simulink model "LowPassFilterTest"  (R2020b)
settings: Solver=FixedStepDiscrete  StartTime=0.0  StopTime=10.0  FixedStep=250e-6  RelTol=1e-3
settings Model: Creator=unix  LastModifiedBy=unix
settings DebuggingCC: IntegerOverflowMsg=error  IntegerSaturationMsg=error

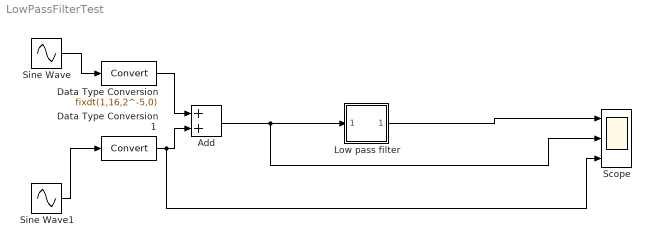
== system LowPassFilterTest ==
  Add : Sum
  Data Type Conversion : DataTypeConversion  OutDataTypeStr=fixdt(1,16,2^-5,0)
  Data Type Conversion1 : DataTypeConversion
  Low pass filter : Subsystem  mask{Value=uint16(200), Gain=250e-6}
      mask prompts: Value "CuttOff Freq."; Gain "Time interval"
      settings: AttributesFormatString=Integration constant %<Gain>
      mask TypeOptions Value: Constant/Value
      mask TypeOptions Gain: Gain/Gain
  Scope : Scope  NumInputPorts=3
  Sine Wave : Sin  Amplitude=12  Frequency=2000  SampleTime=0
  Sine Wave1 : Sin  Amplitude=12  Frequency=100  SampleTime=0
  wires:
  Add/1 -> Scope/2, Low pass filter/1(In1)
  Sine Wave/1 -> Data Type Conversion/1
  Sine Wave1/1 -> Data Type Conversion1/1
  Low pass filter/1(Output) -> Scope/1
  Data Type Conversion/1 -> Add/1
  Data Type Conversion1/1 -> Scope/3, Add/2

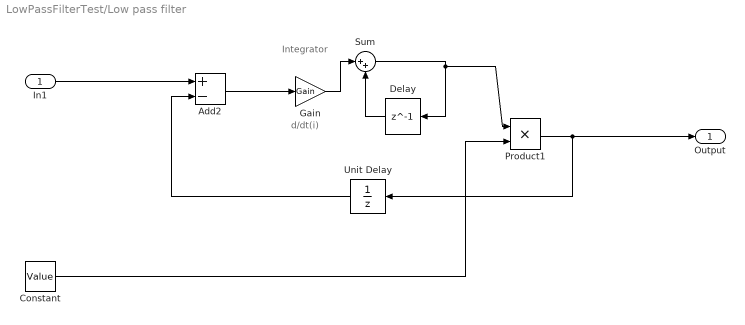
== system LowPassFilterTest/Low pass filter ==
  note: d/dt(i)
  note: Integrator
  In1 : Inport
  Add2 : Sum  Inputs=+-
  Constant : Constant  Value=Value
  Delay : Delay  DelayLength=1  InitialCondition=0
  Gain : Gain  Gain=Gain  ParamDataTypeStr=fixdt(1,16,2^-15,0)  OutMin=-1  OutMax=+1  OutDataTypeStr=fixdt(1,16,2^-14,0)  SaturateOnIntegerOverflow=on
  Product1 : Product  OutDataTypeStr=fixdt(1,16,2^-6,0)
  Sum : Sum  Inputs=|++  OutDataTypeStr=fixdt(1,16,2^-14,0)
  Unit Delay : UnitDelay  SampleTime=-1  HasFrameUpgradeWarning=on
  Output : Outport
  wires:
  Unit Delay/1 -> Add2/2
  Sum/1 -> Product1/1, Delay/1
  Delay/1 -> Sum/2
  Gain/1 -> Sum/1
  Product1/1 -> Unit Delay/1, Output/1
  Add2/1 -> Gain/1
  In1/1 -> Add2/1
  Constant/1 -> Product1/2
